simulink model "Animation3D"  (R2020b)
settings: Solver=VariableStepAuto  StartTime=0.0  StopTime=50  RelTol=1e-3
InitFcn:
  | clear_isnan_data();
libraries: vrlib x1
settings Model: Creator=Mustafa  LastModifiedBy=Mustafa
settings DataIOCC: ReturnWorkspaceOutputs=off
settings DebuggingCC: ArithmeticOperatorsInVariantConditions=warning
settings SFSimCC: SimUseLocalCustomCode=off  CustomCodeUndefinedFunction=UseInterfaceOnly
settings RTWCC: RTWUseLocalCustomCode=off
settings CodeAppCC: StateflowObjectComments=on

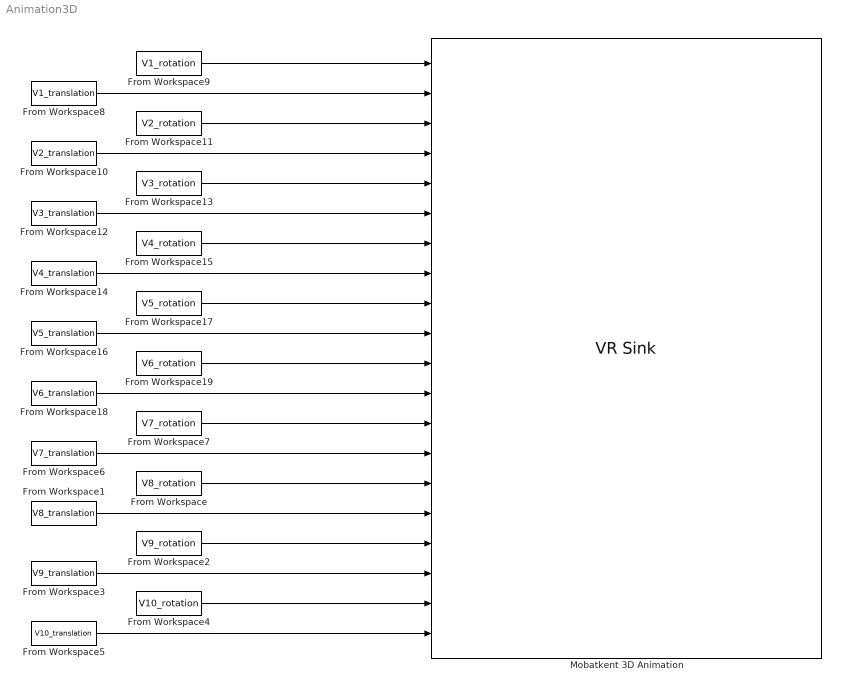
== system Animation3D ==
  From Workspace : FromWorkspace  VariableName=V8_rotation
  From Workspace1 : FromWorkspace  VariableName=V8_translation
  From Workspace10 : FromWorkspace  VariableName=V2_translation
  From Workspace11 : FromWorkspace  VariableName=V2_rotation
  From Workspace12 : FromWorkspace  VariableName=V3_translation
  From Workspace13 : FromWorkspace  VariableName=V3_rotation
  From Workspace14 : FromWorkspace  VariableName=V4_translation
  From Workspace15 : FromWorkspace  VariableName=V4_rotation
  From Workspace16 : FromWorkspace  VariableName=V5_translation
  From Workspace17 : FromWorkspace  VariableName=V5_rotation
  From Workspace18 : FromWorkspace  VariableName=V6_translation
  From Workspace19 : FromWorkspace  VariableName=V6_rotation
  From Workspace2 : FromWorkspace  VariableName=V9_rotation
  From Workspace3 : FromWorkspace  VariableName=V9_translation
  From Workspace4 : FromWorkspace  VariableName=V10_rotation
  From Workspace5 : FromWorkspace  VariableName=V10_translation
  From Workspace6 : FromWorkspace  VariableName=V7_translation
  From Workspace7 : FromWorkspace  VariableName=V7_rotation
  From Workspace8 : FromWorkspace  VariableName=V1_translation
  From Workspace9 : FromWorkspace  VariableName=V1_rotation
  Mobatkent 3D Animation : vrlib/VR Sink  InstantiateOnLoad=on  SampleTime=0.01  ViewEnable=on  RemoteChange=off  RemoteView=off  FieldsWritten=NewCar.rotation.4.1.1.double#NewCar.translation.3.1.1.double#NewCar2.rotation.4.1.1.double#NewCar2.translation.3.1.1.double#NewCar3.rotation.4.1.1.double#NewCar3.translation.3.1.1.double#NewCar4.rotation.4.1.1.double#NewCar4.translation.3.1.1.double#NewCar5.rotation.4.1.1.double#NewCar5.translation.3.1.1.double#NewCar6.rotation.4.1.1.double#NewCar6.translation.3.1.1.double#Car_Mustang.rotation.4.1.1.double#Car_Mustang.translation.3.1.1.double#Fire_Truck.rotation.4.1.1.double#Fire_Truck.translation.3.1.1.double#Car_AR.rotation.4.1.1.double#Car_AR.translation.3.1.1.double#Car_Lotus.rotation.4.1.1.double#Car_Lotus.translation.3.1.1.double  WorldFileName=src\3D Animation\Mobatkent.WRL  AutoView=on  VideoDimensions=[]  AllowVariableSize=off  FigureProperties="{'Position', 'Name', 'Viewpoint', 'CameraBound', 'CameraDirection', 'CameraPosition', 'CameraUpVector', 'ZoomFactor', 'Antialiasing', 'Headlight', 'Lighting', 'NavPanel', 'Sound', 'StatusBar', 'Stereo3D', 'Stereo3DCameraOffset', 'Stereo3DHIT', 'ToolBar', 'Textures', 'Transparency', 'Triad', 'Wireframe', 'NavZones', 'NavMode', 'NavSpeed', 'CaptureFileFormat', 'CaptureFileName', 'Record2DCompressMethod', 'Record2DCompressQuality', 'Record2D', 'Record2DFileName', 'Record2DFPS'; [1.0000000000000000e+00   6.2750000000000000e+01   1.6000000000000000e+03   7.6125000000000000e+02], '', 'Top View', 'on', [0.0000000000000000e+00   0.0000000000000000e+00  -1.0000000000000000e+00], [0.0000000000000000e+00   0.0000000000000000e+00   0.0000000000000000e+00], [0.0000000000000000e+00   1.0000000000000000e+00   0.0000000000000000e+00], [1.0000000000000000e+00], 'on', 'on', 'on', 'halfbar', 'on', 'on', 'off', [1.0000000149011612e-01], [0.0000000000000000e+00], 'on', 'on', 'on', 'none', 'off', 'off', 'fly', 'normal', 'tif', '%f_anim_%n.tif', 'auto', [7.5000000000000000e+01], 'off', '%f_anim_%n.avi', 'auto'}"
  wires:
  From Workspace9/1 -> Mobatkent 3D Animation/1
  From Workspace8/1 -> Mobatkent 3D Animation/2
  From Workspace11/1 -> Mobatkent 3D Animation/3
  From Workspace10/1 -> Mobatkent 3D Animation/4
  From Workspace13/1 -> Mobatkent 3D Animation/5
  From Workspace12/1 -> Mobatkent 3D Animation/6
  From Workspace15/1 -> Mobatkent 3D Animation/7
  From Workspace14/1 -> Mobatkent 3D Animation/8
  From Workspace17/1 -> Mobatkent 3D Animation/9
  From Workspace16/1 -> Mobatkent 3D Animation/10
  From Workspace19/1 -> Mobatkent 3D Animation/11
  From Workspace18/1 -> Mobatkent 3D Animation/12
  From Workspace7/1 -> Mobatkent 3D Animation/13
  From Workspace6/1 -> Mobatkent 3D Animation/14
  From Workspace/1 -> Mobatkent 3D Animation/15
  From Workspace1/1 -> Mobatkent 3D Animation/16
  From Workspace2/1 -> Mobatkent 3D Animation/17
  From Workspace3/1 -> Mobatkent 3D Animation/18
  From Workspace4/1 -> Mobatkent 3D Animation/19
  From Workspace5/1 -> Mobatkent 3D Animation/20
